simulink model "ws1920"  (R2022a)
settings: Solver=FixedStepAuto  StartTime=0.0  StopTime=1  FixedStep=0.001  RelTol=1e-3
values from neighbouring files (symbols this model uses):
  c = 50    [Langmann20mflie.m]
  d = 0.05    [Langmann20mflie.m]
  dL = 5e-6    (= 5e-06)    [Langmann20mflie.m]
  dM = 1.0e-5    (= 1e-05)    [Langmann20mflie.m]
  JL = 2e-5    (= 2e-05)    [Langmann20mflie.m]
  Jm = 0.125e-5    (= 1.25e-06)    [Langmann20mflie.m]
  LM = 1e-3    (= 0.001)    [Langmann20mflie.m]
  ML = 0.25    [Langmann20mflie.m]
  Oi = 2.6e-2    (= 0.026)    [Langmann20mflie.m]
  OM = 0.1125    [Langmann20mflie.m]
  rL = 50.0/1000    (= 0.05)    [Langmann20mflie.m]
  rM = 25/1000    (= 0.025)    [Langmann20mflie.m]
  RM = 1.5    [Langmann20mflie.m]
  Uq0 = 24    [Langmann20mflie.m]
settings Model: Creator=ASUS  LastModifiedBy=ASUS

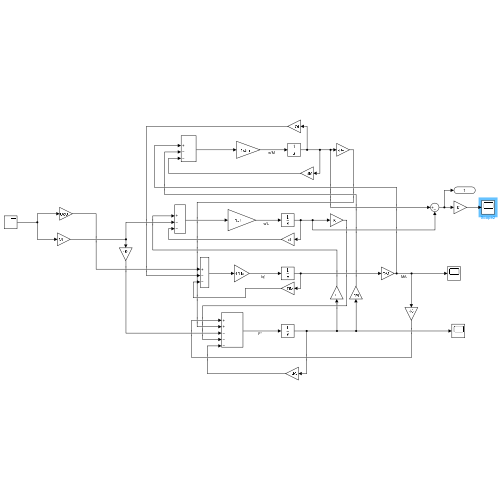
[thumbnail: Simulink's stored preview of the top-level diagram]
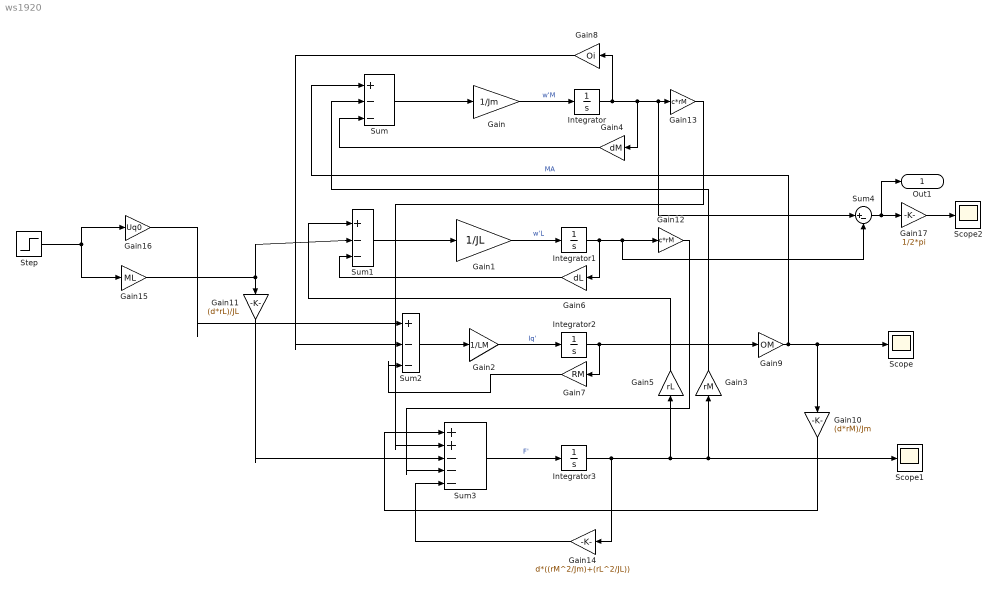
== system ws1920 ==
  Gain : Gain  Gain=1/Jm
  Gain1 : Gain  Gain=1/JL
  Gain10 : Gain  Gain=(d*rM)/Jm
  Gain11 : Gain  Gain=(d*rL)/JL
  Gain12 : Gain  Gain=c*rM
  Gain13 : Gain  Gain=c*rM
  Gain14 : Gain  Gain=d*((rM^2/Jm)+(rL^2/JL))
  Gain15 : Gain  Gain=ML
  Gain16 : Gain  Gain=Uq0
  Gain17 : Gain  Gain=1/2*pi
  Gain2 : Gain  Gain=1/LM
  Gain3 : Gain  Gain=rM
  Gain4 : Gain  Gain=dM
  Gain5 : Gain  Gain=rL
  Gain6 : Gain  Gain=dL
  Gain7 : Gain  Gain=RM
  Gain8 : Gain  Gain=Oi
  Gain9 : Gain  Gain=OM
  Integrator{,1..3} (4 alike) : Integrator
  Scope : Scope
  Scope1 : Scope
  Scope2 : Scope
  Step : Step  Time=0.1  SampleTime=0
  Sum : Sum  Inputs=|+--
  Sum1 : Sum  Inputs=|+--
  Sum2 : Sum  Inputs=|+--
  Sum3 : Sum  Inputs=|++---
  Sum4 : Sum  Inputs=|+-
  Out1 : Outport
  wires:
  Gain/1 -> Integrator/1  "w'M"
  Gain1/1 -> Integrator1/1  "w'L"
  Sum/1 -> Gain/1
  Sum1/1 -> Gain1/1
  Gain2/1 -> Integrator2/1  "Iq'"
  Sum2/1 -> Gain2/1
  Sum3/1 -> Integrator3/1  "F'"
  Integrator3/1 -> Gain14/1, Gain5/1, Gain3/1, Scope1/1
  Gain3/1 -> Sum/2
  Integrator/1 -> Gain8/1, Gain4/1, Sum4/1, Gain13/1
  Gain4/1 -> Sum/3
  Gain5/1 -> Sum1/1
  Integrator1/1 -> Sum4/2, Gain12/1, Gain6/1
  Gain6/1 -> Sum1/3
  Gain15/1 -> Sum1/2, Gain11/1
  Integrator2/1 -> Gain9/1, Gain7/1
  Gain7/1 -> Sum2/3
  Gain8/1 -> Sum2/2
  Gain9/1 -> Sum/1, Scope/1, Gain10/1  "MA"
  Gain10/1 -> Sum3/1
  Gain11/1 -> Sum3/3
  Gain12/1 -> Sum3/4
  Gain13/1 -> Sum3/2
  Gain14/1 -> Sum3/5
  Step/1 -> Gain16/1, Gain15/1
  Gain16/1 -> Sum2/1
  Sum4/1 -> Out1/1, Gain17/1
  Gain17/1 -> Scope2/1
